simulink model "eliminateSSError"  (R2022b)
settings: Solver=VariableStepAuto  StartTime=0.0  StopTime=5  RelTol=1e-3
values from neighbouring files (symbols this model uses):
  Ad = ss_d.A    [ControllerwithDelay.m]    (also in ControllerwithDelay_LQR.m; ControllerwithDelay_PID.m; ControllerwithDelay_SS.m; DiscreteLQControl.m)
  Adaug = [Ad zeros(3,1);-Cd 1]    [ControllerwithDelay_SS.m]    (also in steadyStateError.m = [Ad zeros(size(Ad,1),1); -Cd 0])
  Bd = ss_d.B    [ControllerwithDelay.m]    (also in ControllerwithDelay_LQR.m; ControllerwithDelay_PID.m; ControllerwithDelay_SS.m; DiscreteLQControl.m)
  Bdaug = [Bd; 0]    [ControllerwithDelay_SS.m]    (also in steadyStateError.m)
  Cd = ss_d.C    [ControllerwithDelay.m]    (also in ControllerwithDelay_LQR.m; ControllerwithDelay_PID.m; ControllerwithDelay_SS.m; DiscreteLQControl.m)
  Cdaug = [1 0 0 0]    [ControllerwithDelay_SS.m]    (also in steadyStateError.m = [Cd 0])
  Dd = ss_d.D    [ControllerwithDelay.m]    (also in ControllerwithDelay_LQR.m; ControllerwithDelay_PID.m; ControllerwithDelay_SS.m; DiscreteLQControl.m)
  K2 = place(Adaug,Bdaug,[0.5783+0.2836i,0.5783-0.2836i,0.0150,0.01])    [steadyStateError.m]
undefined symbols (not defined in the file or in its folder): Klqr
libraries: slpidlib x2
settings Model: Creator=1  LastModifiedBy=DAVID CHEN
settings ModelReferenceCC: EnableRefExpFcnMdlSchedulingChecks=on

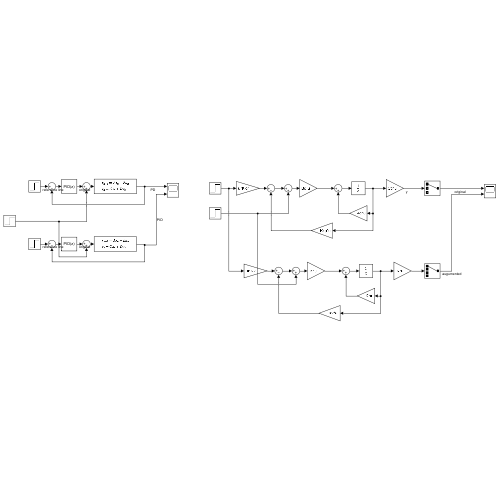
[thumbnail: Simulink's stored preview of the top-level diagram]
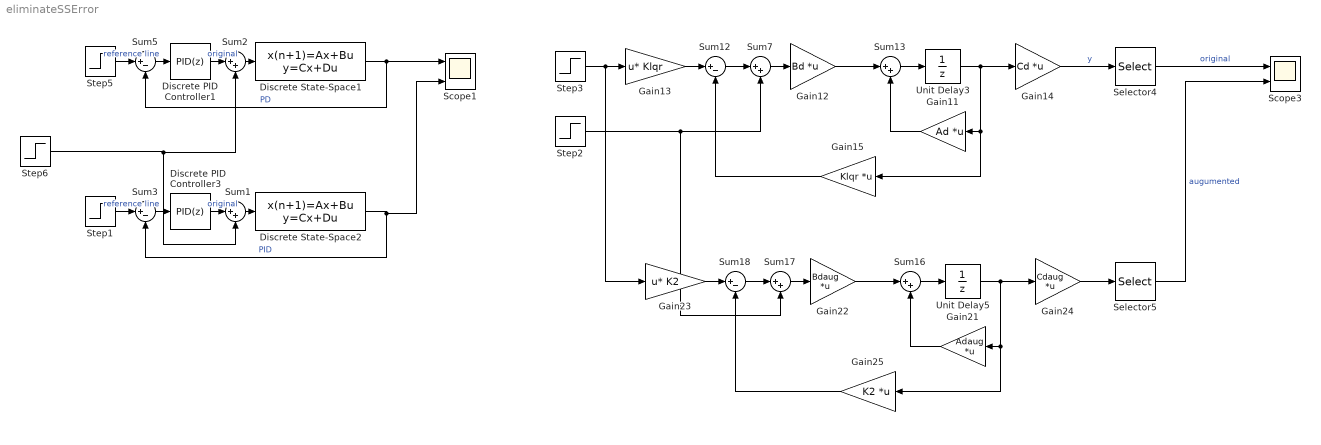
== system eliminateSSError ==
  Discrete PID Controller1 : slpidlib/PID Controller  Controller=PID  Form=Parallel  TimeDomain=Discrete-time  UseExternalTs=off  SampleTime=0.02  IntegratorMethod=Forward Euler  FilterMethod=Forward Euler  ControllerParametersSource=internal  P=0.49  I=0  UseKiTs=off  D=0.08  N=50  UseFilter=on  TunerSelectOption=Transfer Function Based (PID Tuner App)  InitialConditionSource=internal  InitialConditionForIntegrator=0  InitialConditionForFilter=0  DifferentiatorICPrevScaledInput=0  ExternalReset=none  TrackingMode=off  Kt=1  LimitOutput=off  SatLimitsSource=internal  UpperSaturationLimit=inf  LowerSaturationLimit=-inf  LinearizeAsGain=off  AntiWindupMode=none  Kb=1  LimitIntegrator=off  UpperIntegratorSaturationLimit=inf  LowerIntegratorSaturationLimit=-inf  POutMin=[]  POutMax=[]  IOutMin=[]  IOutMax=[]  DOutMin=[]  DOutMax=[]  NOutMin=[]  NOutMax=[]  SumOutMin=[]  SumOutMax=[]  SaturationOutMin=[]  SaturationOutMax=[]  PParamMin=[]  PParamMax=[]  IParamMin=[]  IParamMax=[]  DParamMin=[]  DParamMax=[]  NParamMin=[]  NParamMax=[]  KbParamMin=[]  KbParamMax=[]  KtParamMin=[]  KtParamMax=[]  KbOutMin=[]  KbOutMax=[]  KtOutMin=[]  KtOutMax=[]  IntegratorOutMin=[]  IntegratorOutMax=[]  FilterOutMin=[]  FilterOutMax=[]  SumI1OutMin=[]  SumI1OutMax=[]  SumI2OutMin=[]  SumI2OutMax=[]  SumI3OutMin=[]  SumI3OutMax=[]  SumI4OutMin=[]  SumI4OutMax=[]  SumDOutMin=[]  SumDOutMax=[]  DifferentiatorOutMin=[]  DifferentiatorOutMax=[]  FilterDiffOutCoefMin=[]  FilterDiffOutCoefMax=[]  ReciprocalOutMin=[]  ReciprocalOutMax=[]  SumDenOutMin=[]  SumDenOutMax=[]  SumNumOutMin=[]  SumNumOutMax=[]  DivideOutMin=[]  DivideOutMax=[]  UdiffTsProdOutMin=[]  UdiffTsProdOutMax=[]  NTsProdOutMin=[]  NTsProdOutMax=[]  UintegralTsProdOutMin=[]  UintegralTsProdOutMax=[]  UngainTsProdOutMin=[]  UngainTsProdOutMax=[]  ClampingZeroOutDataTypeStr=Inherit: Inherit via back propagation  ClampingZeroOutMin=[]  ClampingZeroOutMax=[]  FilterDenConstantOutDataTypeStr=Inherit: Inherit via back propagation  FilterDenConstantOutMin=[]  FilterDenConstantOutMax=[]  PCopyOutDataTypeStr=Inherit: Inherit via back propagation  PCopyOutMin=[]  PCopyOutMax=[]  NCopyOutDataTypeStr=Inherit: Inherit via back propagation  NCopyOutMin=[]  NCopyOutMax=[]  IntegratorContinuousStateAttributes=''  IntegratorStateMustResolveToSignalObject=off  IntegratorRTWStateStorageClass=Auto  FilterContinuousStateAttributes=''  FilterStateMustResolveToSignalObject=off  FilterRTWStateStorageClass=Auto  ParallelPVariant=InternalParameters  IdealPVariant=Disabled  IVariant=InternalParameters  DVariant=InternalParameters  IntegratorVariant=Discrete  SatVariant=Disabled  AWVariant=Passthrough  PCopyVariant=Disabled  TRVariant=Disabled  FdbkBlocksVariant=Forward  IdealPFdbkVariant=Disabled  SatFdbkVariant=Disabled  DerivativeFilterVariant=ForwardEulerFilter  NVariant=InternalParameters  NCopyVariant=Disabled  FilterICVariant=InternalICsFilter  IntegratorICVariant=InternalICs  ExternalResetVariant=Disabled  TRSumVariant=Passthrough  SumFdbkVariant=Disabled  SumVariant=Sum_PID  TsampFilterVariant=InternalTs  TsampNgainVariant=Passthrough  TsampIntegralVariant=Passthrough  ExternalSaturationOutDataTypeStr=Inherit: Same as second input
  Discrete PID Controller3 : slpidlib/PID Controller  Controller=PID  Form=Parallel  TimeDomain=Discrete-time  UseExternalTs=off  SampleTime=0.02  IntegratorMethod=Forward Euler  FilterMethod=Forward Euler  ControllerParametersSource=internal  P=0.5  I=0.8  UseKiTs=off  D=0.1  N=50  UseFilter=on  TunerSelectOption=Transfer Function Based (PID Tuner App)  InitialConditionSource=internal  InitialConditionForIntegrator=0  InitialConditionForFilter=0  DifferentiatorICPrevScaledInput=0  ExternalReset=none  TrackingMode=off  Kt=1  LimitOutput=off  SatLimitsSource=internal  UpperSaturationLimit=inf  LowerSaturationLimit=-inf  LinearizeAsGain=off  AntiWindupMode=none  Kb=1  LimitIntegrator=off  UpperIntegratorSaturationLimit=inf  LowerIntegratorSaturationLimit=-inf  POutMin=[]  POutMax=[]  IOutMin=[]  IOutMax=[]  DOutMin=[]  DOutMax=[]  NOutMin=[]  NOutMax=[]  SumOutMin=[]  SumOutMax=[]  SaturationOutMin=[]  SaturationOutMax=[]  PParamMin=[]  PParamMax=[]  IParamMin=[]  IParamMax=[]  DParamMin=[]  DParamMax=[]  NParamMin=[]  NParamMax=[]  KbParamMin=[]  KbParamMax=[]  KtParamMin=[]  KtParamMax=[]  KbOutMin=[]  KbOutMax=[]  KtOutMin=[]  KtOutMax=[]  IntegratorOutMin=[]  IntegratorOutMax=[]  FilterOutMin=[]  FilterOutMax=[]  SumI1OutMin=[]  SumI1OutMax=[]  SumI2OutMin=[]  SumI2OutMax=[]  SumI3OutMin=[]  SumI3OutMax=[]  SumI4OutMin=[]  SumI4OutMax=[]  SumDOutMin=[]  SumDOutMax=[]  DifferentiatorOutMin=[]  DifferentiatorOutMax=[]  FilterDiffOutCoefMin=[]  FilterDiffOutCoefMax=[]  ReciprocalOutMin=[]  ReciprocalOutMax=[]  SumDenOutMin=[]  SumDenOutMax=[]  SumNumOutMin=[]  SumNumOutMax=[]  DivideOutMin=[]  DivideOutMax=[]  UdiffTsProdOutMin=[]  UdiffTsProdOutMax=[]  NTsProdOutMin=[]  NTsProdOutMax=[]  UintegralTsProdOutMin=[]  UintegralTsProdOutMax=[]  UngainTsProdOutMin=[]  UngainTsProdOutMax=[]  ClampingZeroOutDataTypeStr=Inherit: Inherit via back propagation  ClampingZeroOutMin=[]  ClampingZeroOutMax=[]  FilterDenConstantOutDataTypeStr=Inherit: Inherit via back propagation  FilterDenConstantOutMin=[]  FilterDenConstantOutMax=[]  PCopyOutDataTypeStr=Inherit: Inherit via back propagation  PCopyOutMin=[]  PCopyOutMax=[]  NCopyOutDataTypeStr=Inherit: Inherit via back propagation  NCopyOutMin=[]  NCopyOutMax=[]  IntegratorContinuousStateAttributes=''  IntegratorStateMustResolveToSignalObject=off  IntegratorRTWStateStorageClass=Auto  FilterContinuousStateAttributes=''  FilterStateMustResolveToSignalObject=off  FilterRTWStateStorageClass=Auto  ParallelPVariant=InternalParameters  IdealPVariant=Disabled  IVariant=InternalParameters  DVariant=InternalParameters  IntegratorVariant=Discrete  SatVariant=Disabled  AWVariant=Passthrough  PCopyVariant=Disabled  TRVariant=Disabled  FdbkBlocksVariant=Forward  IdealPFdbkVariant=Disabled  SatFdbkVariant=Disabled  DerivativeFilterVariant=ForwardEulerFilter  NVariant=InternalParameters  NCopyVariant=Disabled  FilterICVariant=InternalICsFilter  IntegratorICVariant=InternalICs  ExternalResetVariant=Disabled  TRSumVariant=Passthrough  SumFdbkVariant=Disabled  SumVariant=Sum_PID  TsampFilterVariant=InternalTs  TsampNgainVariant=Passthrough  TsampIntegralVariant=Passthrough  ExternalSaturationOutDataTypeStr=Inherit: Same as second input
  Discrete State-Space1 : DiscreteStateSpace  A=Ad  B=Bd  C=Cd  D=Dd  SampleTime=0.02
  Discrete State-Space2 : DiscreteStateSpace  A=Ad  B=Bd  C=Cd  D=Dd  SampleTime=0.02
  Gain11 : Gain  Gain=Ad  Multiplication=Matrix(K*u)
  Gain12 : Gain  Gain=Bd  Multiplication=Matrix(K*u)
  Gain13 : Gain  Gain=Klqr  Multiplication=Matrix(u*K)
  Gain14 : Gain  Gain=Cd  Multiplication=Matrix(K*u)
  Gain15 : Gain  Gain=Klqr  Multiplication=Matrix(K*u)
  Gain21 : Gain  Gain=Adaug  Multiplication=Matrix(K*u)
  Gain22 : Gain  Gain=Bdaug  Multiplication=Matrix(K*u)
  Gain23 : Gain  Gain=K2  Multiplication=Matrix(u*K)
  Gain24 : Gain  Gain=Cdaug  Multiplication=Matrix(K*u)
  Gain25 : Gain  Gain=K2  Multiplication=Matrix(K*u)
  Scope1 : Scope  NumInputPorts=2
  Scope3 : Scope  NumInputPorts=2
  Selector4 : Selector  InputPortWidth=3  IndexOptions=Index vector (dialog)  Indices=[1]  OutputSizes=1
  Selector5 : Selector  InputPortWidth=4  IndexOptions=Index vector (dialog)  Indices=[1]  OutputSizes=1
  Step1 : Step  Time=0.1  SampleTime=0
  Step2 : Step  SampleTime=0
  Step3 : Step  Time=0  SampleTime=0
  Step5 : Step  Time=0.1  SampleTime=0
  Step6 : Step  SampleTime=0
  Sum{1..2,7,13,16..17} (6 alike) : Sum  Inputs=|++
  Sum{3,5,12,18} (4 alike) : Sum  Inputs=|+-
  Unit Delay3 : UnitDelay  SampleTime=-1  HasFrameUpgradeWarning=on
  Unit Delay5 : UnitDelay  SampleTime=-1  HasFrameUpgradeWarning=on
  wires:
  Step5/1 -> Sum5/1  "reference line"
  Sum5/1 -> Discrete PID Controller1/1
  Discrete State-Space1/1 -> Sum5/2, Scope1/1  "PD"
  Sum2/1 -> Discrete State-Space1/1
  Discrete PID Controller1/1 -> Sum2/1  "original"
  Step6/1 -> Sum1/2, Sum2/2
  Sum1/1 -> Discrete State-Space2/1
  Discrete State-Space2/1 -> Scope1/2, Sum3/2  "PID"
  Sum3/1 -> Discrete PID Controller3/1
  Discrete PID Controller3/1 -> Sum1/1  "original"
  Step1/1 -> Sum3/1  "reference line"
  Sum13/1 -> Unit Delay3/1
  Selector4/1 -> Scope3/1  "original"
  Gain11/1 -> Sum13/2
  Gain14/1 -> Selector4/1  "y"
  Gain13/1 -> Sum12/1
  Unit Delay3/1 -> Gain15/1, Gain11/1, Gain14/1
  Step3/1 -> Gain23/1, Gain13/1
  Gain15/1 -> Sum12/2
  Gain12/1 -> Sum13/1
  Sum12/1 -> Sum7/1
  Sum7/1 -> Gain12/1
  Gain24/1 -> Selector5/1
  Gain22/1 -> Sum16/1
  Unit Delay5/1 -> Gain25/1, Gain21/1, Gain24/1
  Sum17/1 -> Gain22/1
  Gain21/1 -> Sum16/2
  Gain25/1 -> Sum18/2
  Sum18/1 -> Sum17/1
  Gain23/1 -> Sum18/1
  Sum16/1 -> Unit Delay5/1
  Selector5/1 -> Scope3/2  "augumented"
  Step2/1 -> Sum17/2, Sum7/2
